simulink library "isi_correlator_lib"  (Simulink 7.3)
settings: Solver=ode45  SolverMode=SingleTasking  StartTime=0.0  StopTime=10.0  RelTol=1e-3
libraries: xbsIndex_r4 x337, casper_library x37, xps_library x31, isi_correlator_lib x28
(part 2 of 3)

== system isi_correlator_lib/resync ==
  sync_ref : Inport
  sync_in : Inport  Port=2
  data_in : Inport  Port=3
  ASR0 : xbsIndex_r4/Addressable Shift Register  infer_latency=on  depth=2^depth  initVector=[0]  en=off  dbl_ovrd=off  use_behavioral_HDL=off  use_rpm=off  block_type=addrsr
      settings: infoedit="Delay of configurable length.  Any element in the delay line can be addressed and driven onto the output port.<br><br>Hardware notes: Implemented using SRL16s.  If Virtex-4, Virtex-II or Spartan-3 devices are used, multiple SRLC16s are cascaded together."  block_version=10.1.3
  ASR1 : xbsIndex_r4/Addressable Shift Register  infer_latency=on  depth=2^depth  initVector=[0]  en=off  dbl_ovrd=off  use_behavioral_HDL=off  use_rpm=off  block_type=addrsr
      settings: infoedit="Delay of configurable length.  Any element in the delay line can be addressed and driven onto the output port.<br><br>Hardware notes: Implemented using SRL16s.  If Virtex-4, Virtex-II or Spartan-3 devices are used, multiple SRLC16s are cascaded together."  block_version=10.1.3
  Counter : xbsIndex_r4/Counter  cnt_type=Free Running  cnt_to=Inf  operation=Down  start_count=2^depth-1  cnt_by_val=1  arith_type=Unsigned  n_bits=depth  bin_pt=0  load_pin=off  rst=on  en=on  explicit_period=on  period=1  dbl_ovrd=off  use_behavioral_HDL=off  implementation=Fabric  use_rpm=off  block_type=counter
  Inverter0 : xbsIndex_r4/Inverter  en=off  latency=0  dbl_ovrd=off  block_type=inv
  Inverter1 : xbsIndex_r4/Inverter  en=off  latency=0  dbl_ovrd=off  block_type=inv
  Logical1 : xbsIndex_r4/Logical  logical_function=AND  inputs=2  en=off  latency=0  precision=Full  arith_type=Unsigned  n_bits=16  bin_pt=0  align_bp=on  dbl_ovrd=off  block_type=logical
  Register : xbsIndex_r4/Register  init=0  rst=on  en=on  dbl_ovrd=off  block_type=register
  dout : Outport
  aligned : Outport  Port=2
  wires:
  ASR1/1 -> aligned/1
  Inverter0/1 -> Logical1/2
  Logical1/1 -> Register/2
  Register/1 -> ASR1/1, Inverter1/1
  Counter/1 -> ASR1/2, ASR0/2
  Inverter1/1 -> Counter/2
  ASR0/1 -> dout/1
  sync_in/1 -> Register/1, Register/3, Inverter0/1
  sync_ref/1 -> Counter/1, Logical1/1
  data_in/1 -> ASR0/1

== system isi_correlator_lib/saturate ==
  din : Inport  OutDataType=sfix(16)  OutScaling=2^0
  Concat : xbsIndex_r4/Concat  num_inputs=2  dbl_ovrd=off  block_type=concat
      settings: block_version=10.1.3
  Convert : xbsIndex_r4/Convert  arith_type="Signed  (2's comp)"  n_bits=out_bit_width  bin_pt=out_bin_point  quantization=Truncate  overflow=Wrap  latency=2  dbl_ovrd=off  pipeline=off  block_type=convert
      settings: block_version=10.1.3
  Logical : xbsIndex_r4/Logical  logical_function=OR  inputs=2  en=off  latency=0  precision=Full  arith_type=Unsigned  n_bits=8  bin_pt=2  align_bp=on  dbl_ovrd=off  block_type=logical
      settings: xl_area=[0, 0, 0, 0, 0, 0, 0]
  Max : xbsIndex_r4/Constant  arith_type=Signed (2's comp)  const=(2^(out_bit_width-1)-1)/(2^(out_bit_width-1))  n_bits=in_bit_width  bin_pt=in_bin_point  explicit_period=on  period=1  equ=P=C  opselect=C  inp2=PCIN>>17  opr=+  inp1=P  carry=CIN  dbl_ovrd=off  block_type=constant
  Max1 : xbsIndex_r4/Constant  arith_type=Signed (2's comp)  const=(2^(out_bit_width-1)-1)/(2^(out_bit_width-1))  n_bits=out_bit_width  bin_pt=out_bin_point  explicit_period=on  period=1  equ=P=C  opselect=C  inp2=PCIN>>17  opr=+  inp1=P  carry=CIN  dbl_ovrd=off  block_type=constant
  Max2 : xbsIndex_r4/Constant  arith_type=Signed (2's comp)  const=0  n_bits=out_bit_width  bin_pt=out_bin_point  explicit_period=on  period=1  equ=P=C  opselect=C  inp2=PCIN>>17  opr=+  inp1=P  carry=CIN  dbl_ovrd=off  block_type=constant
  Min : xbsIndex_r4/Constant  arith_type=Signed (2's comp)  const=-(2^(out_bit_width - 1) - 1) / 2^(out_bit_width - 1)  n_bits=in_bit_width  bin_pt=in_bin_point  explicit_period=on  period=1  equ=P=C  opselect=C  inp2=PCIN>>17  opr=+  inp1=P  carry=CIN  dbl_ovrd=off  block_type=constant
  Min1 : xbsIndex_r4/Constant  arith_type=Signed (2's comp)  const=-(2^(out_bit_width - 1) - 1) / 2^(out_bit_width - 1)  n_bits=out_bit_width  bin_pt=out_bin_point  explicit_period=on  period=1  equ=P=C  opselect=C  inp2=PCIN>>17  opr=+  inp1=P  carry=CIN  dbl_ovrd=off  block_type=constant
  Mux : xbsIndex_r4/Mux  inputs=4  en=off  latency=0  precision=Full  arith_type="Signed  (2's comp)"  n_bits=8  bin_pt=2  quantization=Truncate  overflow=Wrap  dbl_ovrd=off  block_type=mux
      settings: xl_area=[0, 0, 0, 0, 0, 0, 0]
  Reinterpret_Max : xbsIndex_r4/Reinterpret  force_arith_type=on  arith_type=Unsigned  force_bin_pt=on  bin_pt=0  block_type=reinterpret
      settings: infoedit="Changes signal type without altering the binary representation.   You can changed the signal between signed and unsigned, and relocate the binary point.<P><P>Hardware notes: In hardware this block costs nothing.<P><P>Example:  Suppose the input is 6 bits wide, signed, with 2 fractional bits, and the output is forced to unsigned with 0 fractional bits.  Then an input of -2.0 (1110.00 in binary 2's complement) becomes an output of 56 (111000 in binary)."  block_version=10.1.3
  Reinterpret_Min : xbsIndex_r4/Reinterpret  force_arith_type=on  arith_type=Unsigned  force_bin_pt=on  bin_pt=0  block_type=reinterpret
      settings: infoedit="Changes signal type without altering the binary representation.   You can changed the signal between signed and unsigned, and relocate the binary point.<P><P>Hardware notes: In hardware this block costs nothing.<P><P>Example:  Suppose the input is 6 bits wide, signed, with 2 fractional bits, and the output is forced to unsigned with 0 fractional bits.  Then an input of -2.0 (1110.00 in binary 2's complement) becomes an output of 56 (111000 in binary)."  block_version=10.1.3
  Relational_Max : xbsIndex_r4/Relational  mode=a>b  en=off  latency=2  dbl_ovrd=off  block_type=relational
      settings: xl_area=[0, 0, 0, 0, 0, 0, 0]  block_version=10.1.3
  Relational_Min : xbsIndex_r4/Relational  mode=a<b  en=off  latency=2  dbl_ovrd=off  block_type=relational
      settings: xl_area=[0, 0, 0, 0, 0, 0, 0]  block_version=10.1.3
  dout : Outport  OutDataType=sfix(16)  OutScaling=2^0
  clip : Outport  Port=2  OutDataType=sfix(16)  OutScaling=2^0
  wires:
  Relational_Max/1 -> Logical/1, Reinterpret_Max/1
  Relational_Min/1 -> Logical/2, Reinterpret_Min/1
  Concat/1 -> Mux/1
  Mux/1 -> dout/1
  Logical/1 -> clip/1
  din/1 -> Relational_Min/1, Relational_Max/1, Convert/1
  Max/1 -> Relational_Max/2
  Min/1 -> Relational_Min/2
  Min1/1 -> Mux/3
  Max1/1 -> Mux/4
  Convert/1 -> Mux/2
  Reinterpret_Min/1 -> Concat/2
  Reinterpret_Max/1 -> Concat/1
  Max2/1 -> Mux/5

== system isi_correlator_lib/scale ==
  din : Inport  OutDataType=sfix(16)  OutScaling=2^0
  scale : Inport  Port=2  OutDataType=sfix(16)  OutScaling=2^0
  Logical : xbsIndex_r4/Logical  logical_function=OR  inputs=2  en=off  latency=0  precision=Full  arith_type=Unsigned  n_bits=8  bin_pt=2  align_bp=on  dbl_ovrd=off  block_type=logical
      settings: xl_area=[0, 0, 0, 0, 0, 0, 0]
  Mult_imag : xbsIndex_r4/Mult  precision=Full  arith_type="Signed  (2's comp)"  n_bits=16  bin_pt=14  quantization=Truncate  overflow=Wrap  en=off  latency=3  dbl_ovrd=off  use_behavioral_HDL=off  opt=Speed  use_embedded=on  optimum_pipeline=off  pipeline=on  use_rpm=on  placement_style=Triangular  block_type=mult
      settings: infoedit=Hardware notes: To use the internal pipeline stage of the dedicated multiplier you must select 'Pipeline for maximum performance'.  block_version=10.1.3
  Mult_real : xbsIndex_r4/Mult  precision=Full  arith_type="Signed  (2's comp)"  n_bits=16  bin_pt=14  quantization=Truncate  overflow=Wrap  en=off  latency=3  dbl_ovrd=off  use_behavioral_HDL=off  opt=Speed  use_embedded=on  optimum_pipeline=off  pipeline=on  use_rpm=on  placement_style=Triangular  block_type=mult
      settings: infoedit=Hardware notes: To use the internal pipeline stage of the dedicated multiplier you must select 'Pipeline for maximum performance'.  block_version=10.1.3
  Reinterpret0 : xbsIndex_r4/Reinterpret  force_arith_type=on  arith_type=Unsigned  force_bin_pt=on  bin_pt=0  block_type=reinterpret
      settings: infoedit="Changes signal type without altering the binary representation.   You can changed the signal between signed and unsigned, and relocate the binary point.<P><P>Hardware notes: In hardware this block costs nothing.<P><P>Example:  Suppose the input is 6 bits wide, signed, with 2 fractional bits, and the output is forced to unsigned with 0 fractional bits.  Then an input of -2.0 (1110.00 in binary 2's complement) becomes an output of 56 (111000 in binary)."  block_version=10.1.3
  Reinterpret1 : xbsIndex_r4/Reinterpret  force_arith_type=on  arith_type="Signed  (2's comp)"  force_bin_pt=on  bin_pt=coeff_bin_point  block_type=reinterpret
      settings: infoedit="Changes signal type without altering the binary representation.   You can changed the signal between signed and unsigned, and relocate the binary point.<br><br>Hardware notes: In hardware this block costs nothing.<br><br>Example:  Suppose the input is 6 bits wide, signed, with 2 fractional bits, and the output is forced to unsigned with 0 fractional bits.  Then an input of -2.0 (1110.00 in binary 2's complement) becomes an output of 56 (111000 in binary)."  block_version=10.1.3
  Slice : xbsIndex_r4/Slice  nbits=coeff_bit_width  boolean_output=off  mode=Lower Bit Location + Width  bit1=0  base1=MSB of Input  bit0=0  base0=LSB of Input  dbl_ovrd=off  block_type=slice
      settings: block_version=10.1.3
  c_to_ri : casper_library/Misc/c_to_ri  SystemSampleTime=-1  n_bits=in_bit_width  bin_pt=in_bin_point
      settings: AttributesFormatString=_ r/i
  ri_to_c : casper_library/Misc/ri_to_c  SystemSampleTime=-1
  saturate_imag : isi_correlator_lib/saturate  SystemSampleTime=-1  in_bit_width=in_bit_width + coeff_bit_width  in_bin_point=in_bin_point + coeff_bin_point  out_bit_width=out_bit_width  out_bin_point=out_bin_point
  saturate_real : isi_correlator_lib/saturate  SystemSampleTime=-1  in_bit_width=in_bit_width + coeff_bit_width  in_bin_point=in_bin_point + coeff_bin_point  out_bit_width=out_bit_width  out_bin_point=out_bin_point
  dout : Outport  OutDataType=sfix(16)  OutScaling=2^0
  clip : Outport  Port=2  OutDataType=sfix(16)  OutScaling=2^0
  wires:
  c_to_ri/2 -> Mult_imag/1
  Logical/1 -> clip/1
  Reinterpret1/1 -> Mult_real/2, Mult_imag/2
  scale/1 -> Slice/1
  c_to_ri/1 -> Mult_real/1
  ri_to_c/1 -> dout/1
  Mult_real/1 -> saturate_real/1
  Mult_imag/1 -> saturate_imag/1
  saturate_real/1 -> ri_to_c/1
  saturate_imag/1 -> ri_to_c/2
  saturate_real/2 -> Logical/1
  saturate_imag/2 -> Logical/2
  din/1 -> Reinterpret0/1
  Reinterpret0/1 -> c_to_ri/1
  Slice/1 -> Reinterpret1/1

== system isi_correlator_lib/shuffle ==
  sync : Inport  OutDataType=sfix(16)  OutScaling=2^0
  A : Inport  Port=2  OutDataType=sfix(16)  OutScaling=2^0
  B : Inport  Port=3  OutDataType=sfix(16)  OutScaling=2^0
  C : Inport  Port=4  OutDataType=sfix(16)  OutScaling=2^0
  valid : Inport  Port=5  OutDataType=sfix(16)  OutScaling=2^0
  id : Inport  Port=6  OutDataType=sfix(16)  OutScaling=2^0
  Constant0 : xbsIndex_r4/Constant  arith_type=Unsigned  const=0  n_bits=32  bin_pt=0  explicit_period=on  period=1  equ=P=C  opselect=C  inp2=PCIN>>17  opr=+  inp1=P  carry=CIN  dbl_ovrd=off  block_type=constant
      settings: block_version=10.1.1
  Constant1 : xbsIndex_r4/Constant  arith_type=Unsigned  const=0  n_bits=32  bin_pt=0  explicit_period=on  period=1  equ=P=C  opselect=C  inp2=PCIN>>17  opr=+  inp1=P  carry=CIN  dbl_ovrd=off  block_type=constant
      settings: block_version=10.1.1
  Constant2 : xbsIndex_r4/Constant  arith_type=Unsigned  const=0  n_bits=32  bin_pt=0  explicit_period=on  period=1  equ=P=C  opselect=C  inp2=PCIN>>17  opr=+  inp1=P  carry=CIN  dbl_ovrd=off  block_type=constant
      settings: block_version=10.1.1
  Reinterpret : xbsIndex_r4/Reinterpret  force_arith_type=on  arith_type=Unsigned  force_bin_pt=on  bin_pt=0  block_type=reinterpret
      settings: infoedit="Changes signal type without altering the binary representation.   You can changed the signal between signed and unsigned, and relocate the binary point.<P><P>Hardware notes: In hardware this block costs nothing.<P><P>Example:  Suppose the input is 6 bits wide, signed, with 2 fractional bits, and the output is forced to unsigned with 0 fractional bits.  Then an input of -2.0 (1110.00 in binary 2's complement) becomes an output of 56 (111000 in binary)."  block_version=10.1.1
  Slice : xbsIndex_r4/Slice  nbits=2  boolean_output=off  mode=Lower Bit Location + Width  bit1=0  base1=MSB of Input  bit0=0  base0=LSB of Input  dbl_ovrd=off  block_type=slice
      settings: infoedit="Extracts a given range of bits from each input sample and presents it at the output.  The output type is ordinarily unsigned with binary point at zero, but can be Boolean when the slice is one bit wide.<P><P>Hardware notes: In hardware this block costs nothing."  block_version=10.1.3
  mux_X : xbsIndex_r4/Mux  inputs=4  en=off  latency=latency  precision=Full  arith_type=Unsigned  n_bits=16  bin_pt=14  quantization=Truncate  overflow=Wrap  dbl_ovrd=off  block_type=mux
  mux_Y : xbsIndex_r4/Mux  inputs=4  en=off  latency=latency  precision=Full  arith_type=Unsigned  n_bits=16  bin_pt=14  quantization=Truncate  overflow=Wrap  dbl_ovrd=off  block_type=mux
  mux_Z : xbsIndex_r4/Mux  inputs=4  en=off  latency=latency  precision=Full  arith_type=Unsigned  n_bits=16  bin_pt=14  quantization=Truncate  overflow=Wrap  dbl_ovrd=off  block_type=mux
  sync_delay : xbsIndex_r4/Delay  en=off  latency=latency  dbl_ovrd=off  reg_retiming=off  block_type=delay
  valid_delay : xbsIndex_r4/Delay  en=off  latency=latency  dbl_ovrd=off  reg_retiming=off  block_type=delay
  sync_out : Outport  OutDataType=sfix(16)  OutScaling=2^0
  X : Outport  Port=2  OutDataType=sfix(16)  OutScaling=2^0
  Y : Outport  Port=3  OutDataType=sfix(16)  OutScaling=2^0
  Z : Outport  Port=4  OutDataType=sfix(16)  OutScaling=2^0
  valid_out : Outport  Port=5  OutDataType=sfix(16)  OutScaling=2^0
  wires:
  Constant2/1 -> mux_Z/5
  Constant1/1 -> mux_Y/5
  Constant0/1 -> mux_X/5
  mux_X/1 -> X/1
  mux_Y/1 -> Y/1
  A/1 -> mux_X/2, mux_Y/4, mux_Z/3
  B/1 -> mux_X/3, mux_Y/2, mux_Z/4
  C/1 -> mux_X/4, mux_Y/3, mux_Z/2
  sync/1 -> sync_delay/1
  id/1 -> Slice/1
  sync_delay/1 -> sync_out/1
  mux_Z/1 -> Z/1
  Reinterpret/1 -> mux_X/1, mux_Y/1, mux_Z/1
  Slice/1 -> Reinterpret/1
  valid/1 -> valid_delay/1
  valid_delay/1 -> valid_out/1

== system isi_correlator_lib/sync_gen2 ==
  rst : Inport  OutDataType=sfix(16)  OutScaling=2^0
  AddSub : xbsIndex_r4/AddSub  mode=Subtraction  use_carryin=off  use_carryout=off  en=off  latency=2  precision=Full  arith_type=Unsigned  n_bits=16  bin_pt=14  quantization=Truncate  overflow=Wrap  dbl_ovrd=off  use_behavioral_HDL=off  hw_selection=Fabric  pipelined=off  use_rpm=on  block_type=addsub
      settings: block_version=10.1.3
  Logical1 : xbsIndex_r4/Logical  logical_function=OR  inputs=2  en=off  latency=0  precision=Full  arith_type=Unsigned  n_bits=16  bin_pt=0  align_bp=on  dbl_ovrd=off  block_type=logical
  Mux : xbsIndex_r4/Mux  inputs=2  en=off  latency=0  precision=Full  arith_type=Unsigned  n_bits=16  bin_pt=14  quantization=Truncate  overflow=Wrap  dbl_ovrd=off  block_type=mux
  Relational : xbsIndex_r4/Relational  mode=a>=b  en=off  latency=1  dbl_ovrd=off  block_type=relational
      settings: block_version=10.1.3
  calculated_period : xbsIndex_r4/Constant  arith_type=Unsigned  const=8  n_bits=32  bin_pt=0  explicit_period=on  period=1  equ=P=C  opselect=C  inp2=PCIN>>17  opr=+  inp1=P  carry=CIN  dbl_ovrd=off  block_type=constant
      settings: block_version=10.1.1
  counter : xbsIndex_r4/Counter  cnt_type=Free Running  cnt_to=Inf  operation=Up  start_count=0  cnt_by_val=1  arith_type=Unsigned  n_bits=32  bin_pt=0  load_pin=off  rst=on  en=off  explicit_period=on  period=1  dbl_ovrd=off  use_behavioral_HDL=off  implementation=Fabric  use_rpm=off  block_type=counter
  default_period : Constant  Value=0  OutDataType=sfix(16)  OutScaling=2^0  SampleTime=1
  default_select : Constant  Value=0  OutDataType=sfix(16)  OutScaling=2^0  SampleTime=1
  period : xps_library/software register  Tag=xps:sw_reg  SystemSampleTime=-1  io_dir=From Processor  arith_type=Unsigned  bitwidth=32  bin_pt=0  sample_period=1  gw_name=isi_correlator_lib_sync_gen2_period_user_data_out
  period_offset : xbsIndex_r4/Constant  arith_type=Unsigned  const=3  n_bits=32  bin_pt=0  explicit_period=on  period=1  equ=P=C  opselect=C  inp2=PCIN>>17  opr=+  inp1=P  carry=CIN  dbl_ovrd=off  block_type=constant
      settings: block_version=10.1.1
  posedge : casper_library/Misc/posedge  Tag=Rising Edge Detector  SystemSampleTime=-1
  select : xps_library/software register  Tag=xps:sw_reg  SystemSampleTime=-1  io_dir=From Processor  arith_type=Unsigned  bitwidth=32  bin_pt=0  sample_period=1  gw_name=isi_correlator_lib_sync_gen2_select_user_data_out
  slice_select : xbsIndex_r4/Slice  nbits=1  boolean_output=on  mode=Lower Bit Location + Width  bit1=0  base1=MSB of Input  bit0=0  base0=LSB of Input  dbl_ovrd=off  block_type=slice
      settings: infoedit="Extracts a given range of bits from each input sample and presents it at the output.  The output type is ordinarily unsigned with binary point at zero, but can be Boolean when the slice is one bit wide.<P><P>Hardware notes: In hardware this block costs nothing."  block_version=10.1.3
  sync : Outport  OutDataType=sfix(16)  OutScaling=2^0
  wires:
  rst/1 -> Logical1/2
  Relational/1 -> Logical1/1
  posedge/1 -> sync/1
  Logical1/1 -> counter/1, posedge/1
  counter/1 -> Relational/1
  AddSub/1 -> Relational/2
  period_offset/1 -> AddSub/2
  [period] -> AddSub/1
  default_select/1 -> select/1
  select/1 -> slice_select/1
  default_period/1 -> period/1
  slice_select/1 -> Mux/1
  calculated_period/1 -> Mux/2
  period/1 -> Mux/3
  Mux/1 -> [period]

== system isi_correlator_lib/synced_cntr ==
  sync : Inport
  Counter : xbsIndex_r4/Counter  cnt_type=Free Running  cnt_to=Inf  operation=Up  start_count=0  cnt_by_val=1  arith_type=Unsigned  n_bits=bitwidth  bin_pt=0  load_pin=off  rst=on  en=off  explicit_period=on  period=1  dbl_ovrd=off  use_behavioral_HDL=off  implementation=Fabric  use_rpm=off  block_type=counter
  Inverter : xbsIndex_r4/Inverter  en=off  latency=0  dbl_ovrd=off  block_type=inv
      settings: block_version=11.3
  Logical : xbsIndex_r4/Logical  logical_function=AND  inputs=2  en=off  latency=0  precision=Full  arith_type=Unsigned  n_bits=16  bin_pt=0  align_bp=on  dbl_ovrd=off  block_type=logical
      settings: block_version=11.3
  Slice : xbsIndex_r4/Slice  nbits=1  boolean_output=on  mode=Upper Bit Location + Width  bit1=0  base1=MSB of Input  bit0=0  base0=LSB of Input  dbl_ovrd=off  block_type=slice
      settings: block_version=10.1.1
  negedge : casper_library/Misc/negedge  Tag=Rising Edge Detector  SystemSampleTime=-1
  cnt : Outport
  wires:
  negedge/1 -> Inverter/1
  Logical/1 -> Counter/1
  Inverter/1 -> Logical/2
  Slice/1 -> negedge/1
  sync/1 -> Logical/1
  Counter/1 -> Slice/1, cnt/1

== system isi_correlator_lib/tvg ==
  sync : Inport
  Constant : xbsIndex_r4/Constant  arith_type=Unsigned  const=0  n_bits=32  bin_pt=0  explicit_period=on  period=1  equ=P=C  opselect=C  inp2=PCIN>>17  opr=+  inp1=P  carry=CIN  dbl_ovrd=off  block_type=constant
  Constant1 : xbsIndex_r4/Constant  arith_type=Boolean  const=0  n_bits=32  bin_pt=0  explicit_period=on  period=1  equ=P=C  opselect=C  inp2=PCIN>>17  opr=+  inp1=P  carry=CIN  dbl_ovrd=off  block_type=constant
  bram : xps_library/Shared BRAM  Tag=xps:bram  SystemSampleTime=-1  arith_type="Signed  (2's comp)"  addr_width=11  data_width=32  data_bin_pt=0  init_vals=[1:2^11]  sample_rate=1
  delay3 : xbsIndex_r4/Delay  en=off  latency=1  dbl_ovrd=off  reg_retiming=off  block_type=delay
  synced_cntr : isi_correlator_lib/synced_cntr  SystemSampleTime=-1  bitwidth=addr_width
  sync_out : Outport
  dout : Outport  Port=2
  wires:
  delay3/1 -> sync_out/1
  bram/1 -> dout/1
  synced_cntr/1 -> bram/1
  sync/1 -> delay3/1, synced_cntr/1
  Constant/1 -> bram/2
  Constant1/1 -> bram/3

== system isi_correlator_lib/unclump ==
  sync : Inport
  X : Inport  Port=2
  Y : Inport  Port=3
  Z : Inport  Port=4
  decompressX : isi_correlator_lib/decompress  SystemSampleTime=-1  latency=latency
  decompressY : isi_correlator_lib/decompress  SystemSampleTime=-1  latency=latency
  decompressZ : isi_correlator_lib/decompress  SystemSampleTime=-1  latency=latency
  sync_delay : xbsIndex_r4/Delay  en=off  latency=latency  dbl_ovrd=off  reg_retiming=off  block_type=delay
  sync_delay1 : xbsIndex_r4/Delay  en=off  latency=1  dbl_ovrd=off  reg_retiming=off  block_type=delay
  synced_cntr : isi_correlator_lib/synced_cntr  SystemSampleTime=-1  bitwidth=2
  sync_out : Outport
  XA : Outport  Port=2
  XB : Outport  Port=3
  XC : Outport  Port=4
  YA : Outport  Port=5
  YB : Outport  Port=6
  YC : Outport  Port=7
  ZA : Outport  Port=8
  ZB : Outport  Port=9
  ZC : Outport  Port=10
  wires:
  sync_delay1/1 -> sync_delay/1, synced_cntr/1
  Z/1 -> decompressZ/2
  Y/1 -> decompressY/2
  X/1 -> decompressX/2
  decompressX/1 -> XA/1
  decompressX/2 -> XB/1
  decompressX/3 -> XC/1
  decompressY/1 -> YA/1
  decompressY/2 -> YB/1
  decompressY/3 -> YC/1
  decompressZ/1 -> ZA/1
  decompressZ/2 -> ZB/1
  decompressZ/3 -> ZC/1
  sync/1 -> sync_delay1/1
  sync_delay/1 -> sync_out/1
  synced_cntr/1 -> decompressX/1, decompressZ/1, decompressY/1

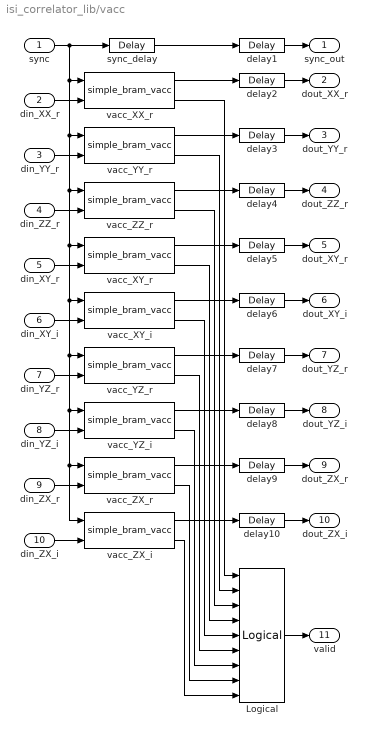
== system isi_correlator_lib/vacc ==
  sync : Inport
  din_XX_r : Inport  Port=2
  din_YY_r : Inport  Port=3
  din_ZZ_r : Inport  Port=4
  din_XY_r : Inport  Port=5
  din_XY_i : Inport  Port=6
  din_YZ_r : Inport  Port=7
  din_YZ_i : Inport  Port=8
  din_ZX_r : Inport  Port=9
  din_ZX_i : Inport  Port=10
  Logical : xbsIndex_r4/Logical  logical_function=AND  inputs=9  en=off  latency=and_delay  precision=Full  arith_type=Unsigned  n_bits=16  bin_pt=0  align_bp=on  dbl_ovrd=off  block_type=logical
  delay{1..10} (10 alike) : xbsIndex_r4/Delay  en=off  latency=and_delay  dbl_ovrd=off  reg_retiming=off  block_type=delay
  sync_delay : xbsIndex_r4/Delay  en=off  latency=2  dbl_ovrd=off  reg_retiming=off  block_type=delay
  vacc_XX_r : casper_library/Accumulators/simple_bram_vacc  SystemSampleTime=-1  n_chans=vector_length  n_bits=out_bit_width  bin_pos=out_bin_point
  vacc_XY_i : casper_library/Accumulators/simple_bram_vacc  SystemSampleTime=-1  n_chans=vector_length  n_bits=out_bit_width  bin_pos=out_bin_point
  vacc_XY_r : casper_library/Accumulators/simple_bram_vacc  SystemSampleTime=-1  n_chans=vector_length  n_bits=out_bit_width  bin_pos=out_bin_point
  vacc_YY_r : casper_library/Accumulators/simple_bram_vacc  SystemSampleTime=-1  n_chans=vector_length  n_bits=out_bit_width  bin_pos=out_bin_point
  vacc_YZ_i : casper_library/Accumulators/simple_bram_vacc  SystemSampleTime=-1  n_chans=vector_length  n_bits=out_bit_width  bin_pos=out_bin_point
  vacc_YZ_r : casper_library/Accumulators/simple_bram_vacc  SystemSampleTime=-1  n_chans=vector_length  n_bits=out_bit_width  bin_pos=out_bin_point
  vacc_ZX_i : casper_library/Accumulators/simple_bram_vacc  SystemSampleTime=-1  n_chans=vector_length  n_bits=out_bit_width  bin_pos=out_bin_point
  vacc_ZX_r : casper_library/Accumulators/simple_bram_vacc  SystemSampleTime=-1  n_chans=vector_length  n_bits=out_bit_width  bin_pos=out_bin_point
  vacc_ZZ_r : casper_library/Accumulators/simple_bram_vacc  SystemSampleTime=-1  n_chans=vector_length  n_bits=out_bit_width  bin_pos=out_bin_point
  sync_out : Outport
  dout_XX_r : Outport  Port=2
  dout_YY_r : Outport  Port=3
  dout_ZZ_r : Outport  Port=4
  dout_XY_r : Outport  Port=5
  dout_XY_i : Outport  Port=6
  dout_YZ_r : Outport  Port=7
  dout_YZ_i : Outport  Port=8
  dout_ZX_r : Outport  Port=9
  dout_ZX_i : Outport  Port=10
  valid : Outport  Port=11
  wires:
  sync/1 -> vacc_ZX_i/1, vacc_ZX_r/1, vacc_YZ_i/1, vacc_YZ_r/1, vacc_XY_i/1, vacc_XY_r/1, vacc_ZZ_r/1, vacc_YY_r/1, vacc_XX_r/1, sync_delay/1
  din_XX_r/1 -> vacc_XX_r/2
  din_YY_r/1 -> vacc_YY_r/2
  din_ZZ_r/1 -> vacc_ZZ_r/2
  din_XY_r/1 -> vacc_XY_r/2
  din_XY_i/1 -> vacc_XY_i/2
  din_YZ_r/1 -> vacc_YZ_r/2
  din_YZ_i/1 -> vacc_YZ_i/2
  din_ZX_r/1 -> vacc_ZX_r/2
  din_ZX_i/1 -> vacc_ZX_i/2
  vacc_XX_r/1 -> delay2/1
  vacc_YY_r/1 -> delay3/1
  vacc_ZZ_r/1 -> delay4/1
  vacc_XY_r/1 -> delay5/1
  vacc_XY_i/1 -> delay6/1
  vacc_YZ_r/1 -> delay7/1
  vacc_YZ_i/1 -> delay8/1
  vacc_ZX_r/1 -> delay9/1
  vacc_ZX_i/1 -> delay10/1
  vacc_XX_r/2 -> Logical/1
  vacc_YY_r/2 -> Logical/2
  vacc_ZZ_r/2 -> Logical/3
  vacc_XY_r/2 -> Logical/4
  vacc_XY_i/2 -> Logical/5
  vacc_YZ_r/2 -> Logical/6
  vacc_YZ_i/2 -> Logical/7
  vacc_ZX_r/2 -> Logical/8
  vacc_ZX_i/2 -> Logical/9
  Logical/1 -> valid/1
  sync_delay/1 -> delay1/1
  delay1/1 -> sync_out/1
  delay2/1 -> dout_XX_r/1
  delay3/1 -> dout_YY_r/1
  delay4/1 -> dout_ZZ_r/1
  delay5/1 -> dout_XY_r/1
  delay6/1 -> dout_XY_i/1
  delay7/1 -> dout_YZ_r/1
  delay8/1 -> dout_YZ_i/1
  delay9/1 -> dout_ZX_r/1
  delay10/1 -> dout_ZX_i/1

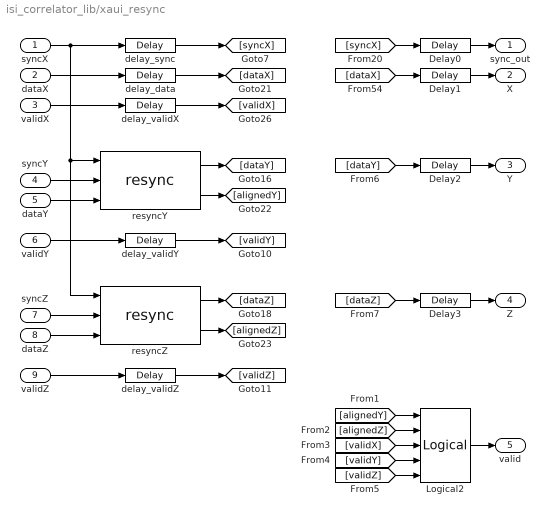
== system isi_correlator_lib/xaui_resync ==
  syncX : Inport  OutDataType=sfix(16)  OutScaling=2^0
  dataX : Inport  Port=2  OutDataType=sfix(16)  OutScaling=2^0
  validX : Inport  Port=3  OutDataType=sfix(16)  OutScaling=2^0
  syncY : Inport  Port=4  OutDataType=sfix(16)  OutScaling=2^0
  dataY : Inport  Port=5  OutDataType=sfix(16)  OutScaling=2^0
  validY : Inport  Port=6  OutDataType=sfix(16)  OutScaling=2^0
  syncZ : Inport  Port=7  OutDataType=sfix(16)  OutScaling=2^0
  dataZ : Inport  Port=8  OutDataType=sfix(16)  OutScaling=2^0
  validZ : Inport  Port=9  OutDataType=sfix(16)  OutScaling=2^0
  Delay{0..3} (4 alike) : xbsIndex_r4/Delay  en=off  latency=logic_latency  dbl_ovrd=off  reg_retiming=off  block_type=delay
  Logical2 : xbsIndex_r4/Logical  logical_function=AND  inputs=5  en=off  latency=logic_latency  precision=Full  arith_type=Unsigned  n_bits=16  bin_pt=0  align_bp=on  dbl_ovrd=off  block_type=logical
  delay_data : xbsIndex_r4/Delay  en=off  latency=2^buffer_depth  dbl_ovrd=off  reg_retiming=off  block_type=delay
  delay_sync : xbsIndex_r4/Delay  en=off  latency=2^buffer_depth  dbl_ovrd=off  reg_retiming=off  block_type=delay
  delay_validX : xbsIndex_r4/Delay  en=off  latency=2^buffer_depth  dbl_ovrd=off  reg_retiming=off  block_type=delay
  delay_validY : xbsIndex_r4/Delay  en=off  latency=2^buffer_depth  dbl_ovrd=off  reg_retiming=off  block_type=delay
  delay_validZ : xbsIndex_r4/Delay  en=off  latency=2^buffer_depth  dbl_ovrd=off  reg_retiming=off  block_type=delay
  resyncY : isi_correlator_lib/resync  SystemSampleTime=-1  depth=buffer_depth
  resyncZ : isi_correlator_lib/resync  SystemSampleTime=-1  depth=buffer_depth
  sync_out : Outport  OutDataType=sfix(16)  OutScaling=2^0
  X : Outport  Port=2  OutDataType=sfix(16)  OutScaling=2^0
  Y : Outport  Port=3  OutDataType=sfix(16)  OutScaling=2^0
  Z : Outport  Port=4  OutDataType=sfix(16)  OutScaling=2^0
  valid : Outport  Port=5  OutDataType=sfix(16)  OutScaling=2^0
  wires:
  [dataX] -> Delay1/1
  Delay1/1 -> X/1
  syncY/1 -> resyncY/2
  dataY/1 -> resyncY/3
  syncZ/1 -> resyncZ/2
  dataZ/1 -> resyncZ/3
  syncX/1 -> resyncY/1, resyncZ/1, delay_sync/1
  dataX/1 -> delay_data/1
  validX/1 -> delay_validX/1
  delay_data/1 -> [dataX]
  delay_sync/1 -> [syncX]
  delay_validX/1 -> [validX]
  [syncX] -> Delay0/1
  Delay0/1 -> sync_out/1
  resyncY/1 -> [dataY]
  resyncY/2 -> [alignedY]
  resyncZ/1 -> [dataZ]
  resyncZ/2 -> [alignedZ]
  delay_validY/1 -> [validY]
  delay_validZ/1 -> [validZ]
  validY/1 -> delay_validY/1
  validZ/1 -> delay_validZ/1
  [alignedY] -> Logical2/1
  [alignedZ] -> Logical2/2
  [validX] -> Logical2/3
  [validY] -> Logical2/4
  [validZ] -> Logical2/5
  Logical2/1 -> valid/1
  [dataZ] -> Delay3/1
  [dataY] -> Delay2/1
  Delay2/1 -> Y/1
  Delay3/1 -> Z/1

== system isi_correlator_lib/capt_adc/data ==
  din0 : Inport
  din1 : Inport  Port=2
  din2 : Inport  Port=3
  din3 : Inport  Port=4
  en : Inport  Port=5
  trig : Inport  Port=6
  Constant : xbsIndex_r4/Constant  arith_type=Boolean  const=1  n_bits=1  bin_pt=0  explicit_period=on  period=1  equ=P=C  opselect=C  inp2=PCIN>>17  opr=+  inp1=P  carry=CIN  dbl_ovrd=off  block_type=constant
      settings: block_version=11.3
  Logical : xbsIndex_r4/Logical  logical_function=AND  inputs=2  en=off  latency=0  precision=Full  arith_type=Unsigned  n_bits=16  bin_pt=0  align_bp=on  dbl_ovrd=off  block_type=logical
      settings: block_version=11.3
  bram{0..3} (4 alike) : xps_library/Shared BRAM  Tag=xps:bram  SystemSampleTime=-1  arith_type=Unsigned  addr_width=addr_width  data_width=32  data_bin_pt=0  init_vals=0  sample_rate=1
  freeze_cntr : casper_library/Misc/freeze_cntr  SystemSampleTime=-1  CounterBits=addr_width
  reinterp{0..3} (4 alike) : xbsIndex_r4/Reinterpret  force_arith_type=on  arith_type=Unsigned  force_bin_pt=on  bin_pt=0  block_type=reinterpret
      settings: infoedit="Changes signal type without altering the binary representation.   You can changed the signal between signed and unsigned, and relocate the binary point.<br><br>Hardware notes: In hardware this block costs nothing.<br><br>Example:  Suppose the input is 6 bits wide, signed, with 2 fractional bits, and the output is forced to unsigned with 0 fractional bits.  Then an input of -2.0 (1110.00 in binary 2's complement) becomes an output of 56 (111000 in binary)."  block_version=11.3
  terminator{0..3} (4 alike) : Terminator
  done : Outport
  wires:
  din0/1 -> reinterp0/1
  reinterp0/1 -> bram0/2
  bram0/1 -> terminator0/1
  din1/1 -> reinterp1/1
  reinterp1/1 -> bram1/2
  bram1/1 -> terminator1/1
  din2/1 -> reinterp2/1
  reinterp2/1 -> bram2/2
  bram2/1 -> terminator2/1
  din3/1 -> reinterp3/1
  reinterp3/1 -> bram3/2
  bram3/1 -> terminator3/1
  freeze_cntr/3 -> done/1
  en/1 -> Logical/1
  trig/1 -> Logical/2
  Constant/1 -> freeze_cntr/1
  Logical/1 -> freeze_cntr/2
  freeze_cntr/1 -> bram0/1, bram1/1, bram2/1, bram3/1
  freeze_cntr/2 -> bram0/3, bram1/3, bram2/3, bram3/3

== system isi_correlator_lib/capt_corr/capt0 ==
  din0 : Inport
  din1 : Inport  Port=2
  din2 : Inport  Port=3
  en : Inport  Port=4
  trig : Inport  Port=5
  Constant : xbsIndex_r4/Constant  arith_type=Boolean  const=1  n_bits=1  bin_pt=0  explicit_period=on  period=1  equ=P=C  opselect=C  inp2=PCIN>>17  opr=+  inp1=P  carry=CIN  dbl_ovrd=off  block_type=constant
      settings: block_version=11.3
  Logical : xbsIndex_r4/Logical  logical_function=AND  inputs=2  en=off  latency=0  precision=Full  arith_type=Unsigned  n_bits=16  bin_pt=0  align_bp=on  dbl_ovrd=off  block_type=logical
      settings: block_version=11.3
  bram0 : xps_library/Shared BRAM  Tag=xps:bram  SystemSampleTime=-1  arith_type=Unsigned  addr_width=addr_width  data_width=32  data_bin_pt=0  init_vals=0  sample_rate=1
  bram1 : xps_library/Shared BRAM  Tag=xps:bram  SystemSampleTime=-1  arith_type=Unsigned  addr_width=addr_width  data_width=32  data_bin_pt=0  init_vals=0  sample_rate=1
  bram2 : xps_library/Shared BRAM  Tag=xps:bram  SystemSampleTime=-1  arith_type=Unsigned  addr_width=addr_width  data_width=32  data_bin_pt=0  init_vals=0  sample_rate=1
  freeze_cntr : casper_library/Misc/freeze_cntr  SystemSampleTime=-1  CounterBits=addr_width
  reinterp0 : xbsIndex_r4/Reinterpret  force_arith_type=on  arith_type=Unsigned  force_bin_pt=on  bin_pt=0  block_type=reinterpret
      settings: infoedit="Changes signal type without altering the binary representation.   You can changed the signal between signed and unsigned, and relocate the binary point.<br><br>Hardware notes: In hardware this block costs nothing.<br><br>Example:  Suppose the input is 6 bits wide, signed, with 2 fractional bits, and the output is forced to unsigned with 0 fractional bits.  Then an input of -2.0 (1110.00 in binary 2's complement) becomes an output of 56 (111000 in binary)."  block_version=11.3
  reinterp1 : xbsIndex_r4/Reinterpret  force_arith_type=on  arith_type=Unsigned  force_bin_pt=on  bin_pt=0  block_type=reinterpret
      settings: infoedit="Changes signal type without altering the binary representation.   You can changed the signal between signed and unsigned, and relocate the binary point.<br><br>Hardware notes: In hardware this block costs nothing.<br><br>Example:  Suppose the input is 6 bits wide, signed, with 2 fractional bits, and the output is forced to unsigned with 0 fractional bits.  Then an input of -2.0 (1110.00 in binary 2's complement) becomes an output of 56 (111000 in binary)."  block_version=11.3
  reinterp2 : xbsIndex_r4/Reinterpret  force_arith_type=on  arith_type=Unsigned  force_bin_pt=on  bin_pt=0  block_type=reinterpret
      settings: infoedit="Changes signal type without altering the binary representation.   You can changed the signal between signed and unsigned, and relocate the binary point.<br><br>Hardware notes: In hardware this block costs nothing.<br><br>Example:  Suppose the input is 6 bits wide, signed, with 2 fractional bits, and the output is forced to unsigned with 0 fractional bits.  Then an input of -2.0 (1110.00 in binary 2's complement) becomes an output of 56 (111000 in binary)."  block_version=11.3
  terminator0 : Terminator
  terminator1 : Terminator
  terminator2 : Terminator
  done : Outport
  wires:
  din0/1 -> reinterp0/1
  reinterp0/1 -> bram0/2
  bram0/1 -> terminator0/1
  din1/1 -> reinterp1/1
  reinterp1/1 -> bram1/2
  bram1/1 -> terminator1/1
  din2/1 -> reinterp2/1
  reinterp2/1 -> bram2/2
  bram2/1 -> terminator2/1
  freeze_cntr/3 -> done/1
  en/1 -> Logical/1
  trig/1 -> Logical/2
  Constant/1 -> freeze_cntr/1
  Logical/1 -> freeze_cntr/2
  freeze_cntr/1 -> bram0/1, bram1/1, bram2/1
  freeze_cntr/2 -> bram0/3, bram1/3, bram2/3

== system isi_correlator_lib/capt_corr/capt1 ==
  din0 : Inport
  din1 : Inport  Port=2
  din2 : Inport  Port=3
  en : Inport  Port=4
  trig : Inport  Port=5
  Constant : xbsIndex_r4/Constant  arith_type=Boolean  const=1  n_bits=1  bin_pt=0  explicit_period=on  period=1  equ=P=C  opselect=C  inp2=PCIN>>17  opr=+  inp1=P  carry=CIN  dbl_ovrd=off  block_type=constant
      settings: block_version=11.3
  Logical : xbsIndex_r4/Logical  logical_function=AND  inputs=2  en=off  latency=0  precision=Full  arith_type=Unsigned  n_bits=16  bin_pt=0  align_bp=on  dbl_ovrd=off  block_type=logical
      settings: block_version=11.3
  bram0 : xps_library/Shared BRAM  Tag=xps:bram  SystemSampleTime=-1  arith_type=Unsigned  addr_width=addr_width  data_width=32  data_bin_pt=0  init_vals=0  sample_rate=1
  bram1 : xps_library/Shared BRAM  Tag=xps:bram  SystemSampleTime=-1  arith_type=Unsigned  addr_width=addr_width  data_width=32  data_bin_pt=0  init_vals=0  sample_rate=1
  bram2 : xps_library/Shared BRAM  Tag=xps:bram  SystemSampleTime=-1  arith_type=Unsigned  addr_width=addr_width  data_width=32  data_bin_pt=0  init_vals=0  sample_rate=1
  freeze_cntr : casper_library/Misc/freeze_cntr  SystemSampleTime=-1  CounterBits=addr_width
  reinterp0 : xbsIndex_r4/Reinterpret  force_arith_type=on  arith_type=Unsigned  force_bin_pt=on  bin_pt=0  block_type=reinterpret
      settings: infoedit="Changes signal type without altering the binary representation.   You can changed the signal between signed and unsigned, and relocate the binary point.<br><br>Hardware notes: In hardware this block costs nothing.<br><br>Example:  Suppose the input is 6 bits wide, signed, with 2 fractional bits, and the output is forced to unsigned with 0 fractional bits.  Then an input of -2.0 (1110.00 in binary 2's complement) becomes an output of 56 (111000 in binary)."  block_version=11.3
  reinterp1 : xbsIndex_r4/Reinterpret  force_arith_type=on  arith_type=Unsigned  force_bin_pt=on  bin_pt=0  block_type=reinterpret
      settings: infoedit="Changes signal type without altering the binary representation.   You can changed the signal between signed and unsigned, and relocate the binary point.<br><br>Hardware notes: In hardware this block costs nothing.<br><br>Example:  Suppose the input is 6 bits wide, signed, with 2 fractional bits, and the output is forced to unsigned with 0 fractional bits.  Then an input of -2.0 (1110.00 in binary 2's complement) becomes an output of 56 (111000 in binary)."  block_version=11.3
  reinterp2 : xbsIndex_r4/Reinterpret  force_arith_type=on  arith_type=Unsigned  force_bin_pt=on  bin_pt=0  block_type=reinterpret
      settings: infoedit="Changes signal type without altering the binary representation.   You can changed the signal between signed and unsigned, and relocate the binary point.<br><br>Hardware notes: In hardware this block costs nothing.<br><br>Example:  Suppose the input is 6 bits wide, signed, with 2 fractional bits, and the output is forced to unsigned with 0 fractional bits.  Then an input of -2.0 (1110.00 in binary 2's complement) becomes an output of 56 (111000 in binary)."  block_version=11.3
  terminator0 : Terminator
  terminator1 : Terminator
  terminator2 : Terminator
  terminator_done : Terminator
  wires:
  din0/1 -> reinterp0/1
  reinterp0/1 -> bram0/2
  bram0/1 -> terminator0/1
  din1/1 -> reinterp1/1
  reinterp1/1 -> bram1/2
  bram1/1 -> terminator1/1
  din2/1 -> reinterp2/1
  reinterp2/1 -> bram2/2
  bram2/1 -> terminator2/1
  freeze_cntr/3 -> terminator_done/1
  en/1 -> Logical/1
  trig/1 -> Logical/2
  Constant/1 -> freeze_cntr/1
  Logical/1 -> freeze_cntr/2
  freeze_cntr/1 -> bram0/1, bram1/1, bram2/1
  freeze_cntr/2 -> bram0/3, bram1/3, bram2/3

== system isi_correlator_lib/capt_corr/capt2 ==
  din0 : Inport
  din1 : Inport  Port=2
  din2 : Inport  Port=3
  en : Inport  Port=4
  trig : Inport  Port=5
  Constant : xbsIndex_r4/Constant  arith_type=Boolean  const=1  n_bits=1  bin_pt=0  explicit_period=on  period=1  equ=P=C  opselect=C  inp2=PCIN>>17  opr=+  inp1=P  carry=CIN  dbl_ovrd=off  block_type=constant
      settings: block_version=11.3
  Logical : xbsIndex_r4/Logical  logical_function=AND  inputs=2  en=off  latency=0  precision=Full  arith_type=Unsigned  n_bits=16  bin_pt=0  align_bp=on  dbl_ovrd=off  block_type=logical
      settings: block_version=11.3
  bram0 : xps_library/Shared BRAM  Tag=xps:bram  SystemSampleTime=-1  arith_type=Unsigned  addr_width=addr_width  data_width=32  data_bin_pt=0  init_vals=0  sample_rate=1
  bram1 : xps_library/Shared BRAM  Tag=xps:bram  SystemSampleTime=-1  arith_type=Unsigned  addr_width=addr_width  data_width=32  data_bin_pt=0  init_vals=0  sample_rate=1
  bram2 : xps_library/Shared BRAM  Tag=xps:bram  SystemSampleTime=-1  arith_type=Unsigned  addr_width=addr_width  data_width=32  data_bin_pt=0  init_vals=0  sample_rate=1
  freeze_cntr : casper_library/Misc/freeze_cntr  SystemSampleTime=-1  CounterBits=addr_width
  reinterp0 : xbsIndex_r4/Reinterpret  force_arith_type=on  arith_type=Unsigned  force_bin_pt=on  bin_pt=0  block_type=reinterpret
      settings: infoedit="Changes signal type without altering the binary representation.   You can changed the signal between signed and unsigned, and relocate the binary point.<br><br>Hardware notes: In hardware this block costs nothing.<br><br>Example:  Suppose the input is 6 bits wide, signed, with 2 fractional bits, and the output is forced to unsigned with 0 fractional bits.  Then an input of -2.0 (1110.00 in binary 2's complement) becomes an output of 56 (111000 in binary)."  block_version=11.3
  reinterp1 : xbsIndex_r4/Reinterpret  force_arith_type=on  arith_type=Unsigned  force_bin_pt=on  bin_pt=0  block_type=reinterpret
      settings: infoedit="Changes signal type without altering the binary representation.   You can changed the signal between signed and unsigned, and relocate the binary point.<br><br>Hardware notes: In hardware this block costs nothing.<br><br>Example:  Suppose the input is 6 bits wide, signed, with 2 fractional bits, and the output is forced to unsigned with 0 fractional bits.  Then an input of -2.0 (1110.00 in binary 2's complement) becomes an output of 56 (111000 in binary)."  block_version=11.3
  reinterp2 : xbsIndex_r4/Reinterpret  force_arith_type=on  arith_type=Unsigned  force_bin_pt=on  bin_pt=0  block_type=reinterpret
      settings: infoedit="Changes signal type without altering the binary representation.   You can changed the signal between signed and unsigned, and relocate the binary point.<br><br>Hardware notes: In hardware this block costs nothing.<br><br>Example:  Suppose the input is 6 bits wide, signed, with 2 fractional bits, and the output is forced to unsigned with 0 fractional bits.  Then an input of -2.0 (1110.00 in binary 2's complement) becomes an output of 56 (111000 in binary)."  block_version=11.3
  terminator0 : Terminator
  terminator1 : Terminator
  terminator2 : Terminator
  terminator_done : Terminator
  wires:
  din0/1 -> reinterp0/1
  reinterp0/1 -> bram0/2
  bram0/1 -> terminator0/1
  din1/1 -> reinterp1/1
  reinterp1/1 -> bram1/2
  bram1/1 -> terminator1/1
  din2/1 -> reinterp2/1
  reinterp2/1 -> bram2/2
  bram2/1 -> terminator2/1
  freeze_cntr/3 -> terminator_done/1
  en/1 -> Logical/1
  trig/1 -> Logical/2
  Constant/1 -> freeze_cntr/1
  Logical/1 -> freeze_cntr/2
  freeze_cntr/1 -> bram0/1, bram1/1, bram2/1
  freeze_cntr/2 -> bram0/3, bram1/3, bram2/3

== system isi_correlator_lib/capt_fft/lsb ==
  din0 : Inport
  din1 : Inport  Port=2
  din2 : Inport  Port=3
  din3 : Inport  Port=4
  en : Inport  Port=5
  trig : Inport  Port=6
  Constant : xbsIndex_r4/Constant  arith_type=Boolean  const=1  n_bits=1  bin_pt=0  explicit_period=on  period=1  equ=P=C  opselect=C  inp2=PCIN>>17  opr=+  inp1=P  carry=CIN  dbl_ovrd=off  block_type=constant
      settings: block_version=11.3
  Logical : xbsIndex_r4/Logical  logical_function=AND  inputs=2  en=off  latency=0  precision=Full  arith_type=Unsigned  n_bits=16  bin_pt=0  align_bp=on  dbl_ovrd=off  block_type=logical
      settings: block_version=11.3
  bram{0..3} (4 alike) : xps_library/Shared BRAM  Tag=xps:bram  SystemSampleTime=-1  arith_type=Unsigned  addr_width=addr_width  data_width=32  data_bin_pt=0  init_vals=0  sample_rate=1
  freeze_cntr : casper_library/Misc/freeze_cntr  SystemSampleTime=-1  CounterBits=addr_width
  reinterp{0..3} (4 alike) : xbsIndex_r4/Reinterpret  force_arith_type=on  arith_type=Unsigned  force_bin_pt=on  bin_pt=0  block_type=reinterpret
      settings: infoedit="Changes signal type without altering the binary representation.   You can changed the signal between signed and unsigned, and relocate the binary point.<br><br>Hardware notes: In hardware this block costs nothing.<br><br>Example:  Suppose the input is 6 bits wide, signed, with 2 fractional bits, and the output is forced to unsigned with 0 fractional bits.  Then an input of -2.0 (1110.00 in binary 2's complement) becomes an output of 56 (111000 in binary)."  block_version=11.3
  terminator{0..3} (4 alike) : Terminator
  terminator_done : Terminator
  wires:
  din0/1 -> reinterp0/1
  reinterp0/1 -> bram0/2
  bram0/1 -> terminator0/1
  din1/1 -> reinterp1/1
  reinterp1/1 -> bram1/2
  bram1/1 -> terminator1/1
  din2/1 -> reinterp2/1
  reinterp2/1 -> bram2/2
  bram2/1 -> terminator2/1
  din3/1 -> reinterp3/1
  reinterp3/1 -> bram3/2
  bram3/1 -> terminator3/1
  freeze_cntr/3 -> terminator_done/1
  en/1 -> Logical/1
  trig/1 -> Logical/2
  Constant/1 -> freeze_cntr/1
  Logical/1 -> freeze_cntr/2
  freeze_cntr/1 -> bram0/1, bram1/1, bram2/1, bram3/1
  freeze_cntr/2 -> bram0/3, bram1/3, bram2/3, bram3/3

== system isi_correlator_lib/capt_fft/msb ==
  din0 : Inport
  din1 : Inport  Port=2
  din2 : Inport  Port=3
  din3 : Inport  Port=4
  en : Inport  Port=5
  trig : Inport  Port=6
  Constant : xbsIndex_r4/Constant  arith_type=Boolean  const=1  n_bits=1  bin_pt=0  explicit_period=on  period=1  equ=P=C  opselect=C  inp2=PCIN>>17  opr=+  inp1=P  carry=CIN  dbl_ovrd=off  block_type=constant
      settings: block_version=11.3
  Logical : xbsIndex_r4/Logical  logical_function=AND  inputs=2  en=off  latency=0  precision=Full  arith_type=Unsigned  n_bits=16  bin_pt=0  align_bp=on  dbl_ovrd=off  block_type=logical
      settings: block_version=11.3
  bram{0..3} (4 alike) : xps_library/Shared BRAM  Tag=xps:bram  SystemSampleTime=-1  arith_type=Unsigned  addr_width=addr_width  data_width=32  data_bin_pt=0  init_vals=0  sample_rate=1
  freeze_cntr : casper_library/Misc/freeze_cntr  SystemSampleTime=-1  CounterBits=addr_width
  reinterp{0..3} (4 alike) : xbsIndex_r4/Reinterpret  force_arith_type=on  arith_type=Unsigned  force_bin_pt=on  bin_pt=0  block_type=reinterpret
      settings: infoedit="Changes signal type without altering the binary representation.   You can changed the signal between signed and unsigned, and relocate the binary point.<br><br>Hardware notes: In hardware this block costs nothing.<br><br>Example:  Suppose the input is 6 bits wide, signed, with 2 fractional bits, and the output is forced to unsigned with 0 fractional bits.  Then an input of -2.0 (1110.00 in binary 2's complement) becomes an output of 56 (111000 in binary)."  block_version=11.3
  terminator{0..3} (4 alike) : Terminator
  done : Outport
  wires:
  din0/1 -> reinterp0/1
  reinterp0/1 -> bram0/2
  bram0/1 -> terminator0/1
  din1/1 -> reinterp1/1
  reinterp1/1 -> bram1/2
  bram1/1 -> terminator1/1
  din2/1 -> reinterp2/1
  reinterp2/1 -> bram2/2
  bram2/1 -> terminator2/1
  din3/1 -> reinterp3/1
  reinterp3/1 -> bram3/2
  bram3/1 -> terminator3/1
  freeze_cntr/3 -> done/1
  en/1 -> Logical/1
  trig/1 -> Logical/2
  Constant/1 -> freeze_cntr/1
  Logical/1 -> freeze_cntr/2
  freeze_cntr/1 -> bram0/1, bram1/1, bram2/1, bram3/1
  freeze_cntr/2 -> bram0/3, bram1/3, bram2/3, bram3/3

== system isi_correlator_lib/capt_xaui/capt0 ==
  din0 : Inport
  din1 : Inport  Port=2
  din2 : Inport  Port=3
  en : Inport  Port=4
  trig : Inport  Port=5
  Constant : xbsIndex_r4/Constant  arith_type=Boolean  const=1  n_bits=1  bin_pt=0  explicit_period=on  period=1  equ=P=C  opselect=C  inp2=PCIN>>17  opr=+  inp1=P  carry=CIN  dbl_ovrd=off  block_type=constant
      settings: block_version=11.3
  Logical : xbsIndex_r4/Logical  logical_function=AND  inputs=2  en=off  latency=0  precision=Full  arith_type=Unsigned  n_bits=16  bin_pt=0  align_bp=on  dbl_ovrd=off  block_type=logical
      settings: block_version=11.3
  bram0 : xps_library/Shared BRAM  Tag=xps:bram  SystemSampleTime=-1  arith_type=Unsigned  addr_width=addr_width  data_width=32  data_bin_pt=0  init_vals=0  sample_rate=1
  bram1 : xps_library/Shared BRAM  Tag=xps:bram  SystemSampleTime=-1  arith_type=Unsigned  addr_width=addr_width  data_width=32  data_bin_pt=0  init_vals=0  sample_rate=1
  bram2 : xps_library/Shared BRAM  Tag=xps:bram  SystemSampleTime=-1  arith_type=Unsigned  addr_width=addr_width  data_width=32  data_bin_pt=0  init_vals=0  sample_rate=1
  freeze_cntr : casper_library/Misc/freeze_cntr  SystemSampleTime=-1  CounterBits=addr_width
  reinterp0 : xbsIndex_r4/Reinterpret  force_arith_type=on  arith_type=Unsigned  force_bin_pt=on  bin_pt=0  block_type=reinterpret
      settings: infoedit="Changes signal type without altering the binary representation.   You can changed the signal between signed and unsigned, and relocate the binary point.<br><br>Hardware notes: In hardware this block costs nothing.<br><br>Example:  Suppose the input is 6 bits wide, signed, with 2 fractional bits, and the output is forced to unsigned with 0 fractional bits.  Then an input of -2.0 (1110.00 in binary 2's complement) becomes an output of 56 (111000 in binary)."  block_version=11.3
  reinterp1 : xbsIndex_r4/Reinterpret  force_arith_type=on  arith_type=Unsigned  force_bin_pt=on  bin_pt=0  block_type=reinterpret
      settings: infoedit="Changes signal type without altering the binary representation.   You can changed the signal between signed and unsigned, and relocate the binary point.<br><br>Hardware notes: In hardware this block costs nothing.<br><br>Example:  Suppose the input is 6 bits wide, signed, with 2 fractional bits, and the output is forced to unsigned with 0 fractional bits.  Then an input of -2.0 (1110.00 in binary 2's complement) becomes an output of 56 (111000 in binary)."  block_version=11.3
  reinterp2 : xbsIndex_r4/Reinterpret  force_arith_type=on  arith_type=Unsigned  force_bin_pt=on  bin_pt=0  block_type=reinterpret
      settings: infoedit="Changes signal type without altering the binary representation.   You can changed the signal between signed and unsigned, and relocate the binary point.<br><br>Hardware notes: In hardware this block costs nothing.<br><br>Example:  Suppose the input is 6 bits wide, signed, with 2 fractional bits, and the output is forced to unsigned with 0 fractional bits.  Then an input of -2.0 (1110.00 in binary 2's complement) becomes an output of 56 (111000 in binary)."  block_version=11.3
  terminator0 : Terminator
  terminator1 : Terminator
  terminator2 : Terminator
  done : Outport
  wires:
  din0/1 -> reinterp0/1
  reinterp0/1 -> bram0/2
  bram0/1 -> terminator0/1
  din1/1 -> reinterp1/1
  reinterp1/1 -> bram1/2
  bram1/1 -> terminator1/1
  din2/1 -> reinterp2/1
  reinterp2/1 -> bram2/2
  bram2/1 -> terminator2/1
  freeze_cntr/3 -> done/1
  en/1 -> Logical/1
  trig/1 -> Logical/2
  Constant/1 -> freeze_cntr/1
  Logical/1 -> freeze_cntr/2
  freeze_cntr/1 -> bram0/1, bram1/1, bram2/1
  freeze_cntr/2 -> bram0/3, bram1/3, bram2/3
